simulink model "KeplerianPropagator_Basic"  (R2017b)
settings: Solver=ode3  StartTime=0.0  StopTime=stopTime  FixedStep=stepSize  MaxStep=100  RelTol=1e-3  EnableMultiTasking=on
values from neighbouring files (symbols this model uses):
  a = a_d    (= 6782.423)    [AA279D_hw4.m]    (also in AA279D_hw4_v2.m = 7500; SCHAUBprop.m = oe(1); TLE_Reader.m = (mu/n^2)^(1/3); keplerUniversal.m = 1./alpha(idx))
  e = 0    [AA279D_PSET3.m]    (also in AA279D_PSET4.m = 0.1; AA279D_hw4.m = 0.7; AA279D_hw4_v2.m = 0.1; SCHAUBprop.m = oe(2))
  i = i_d    [AA279D_hw4.m]    (also in SCHAUBprop.m = oe(3); dv_hardcod.m = cin+1; dv_timer.m = cin+1; oe2roe.m = oe_c(3))
  M0 = M    [AA279D_FINAL.m]    (also in AA279D_PSET1.m; AA279D_PSET2.m; AA279D_PSET2_a_change.m; AA279D_PSET3.m)
  n = n_D    [AA279D_hw4.m]    (also in AA279D_hw4_v2.m = sqrt(mu/a^3); AA279D_hw5_dv.m = sqrt(mu/at^3); OE2ECI.m = sqrt(mu/a^3); TLE_Reader.m = revs_per_day*2*pi/(24*3600))
  RAAN = 0    [AA279D_FINAL.m]    (also in AA279D_hw4_v2.m = deg2rad(358.1559); TLE_Reader.m = L3(1,4); test_space.mat = 331.1221)
  tol = 10^-5    (= 1e-05)    [AA279D_FINAL.m]    (also in AA279D_PSET1.m; AA279D_PSET2.m; AA279D_PSET2_a_change.m; AA279D_PSET3.m)
  w = 0    [AA279D_FINAL.m]    (also in AA279D_hw4.m = w_d; AA279D_hw4_v2.m = deg2rad(358.729); SCHAUBprop.m = oe(5); TLE_Reader.m = L3(1,6))
libraries: simulink_extras x4
settings Model: Creator=Lloyd  LastModifiedBy=cwcovert
settings DataIOCC: LimitDataPoints=on  SaveFormat=Array
settings OptimizationCC: LifeSpan=inf
settings DebuggingCC: SolverPrmCheckMsg=warning  SFUnexpectedBacktrackingDiag=warning  SFNoUnconditionalDefaultTransitionDiag=warning  SFExecutionAtInitializationDiag=none
settings HardwareCC: ProdBitPerPointer=32  ProdBitPerSizeT=32  ProdBitPerPtrDiffT=32  ProdLargestAtomicFloat=None  ProdIntDivRoundTo=Undefined  ProdEndianess=Unspecified  ProdWordSize=32  ProdHWDeviceType=32-bit Generic
settings ModelReferenceCC: PropagateSignalLabelsOutOfModel=off
settings CodeAppCC: StateflowObjectComments=on
settings GRTTargetCC: TargetLangStandard=C89/C90 (ANSI)  GeneratePreprocessorConditionals=Disable all
settings ConfigComp: CovMetricSettings=dw  CovHtmlReporting=on  CovSaveCumulativeToWorkspaceVar=on  CovSaveSingleToWorkspaceVar=on  CovExternalEMLEnable=off  CovSFcnEnable=off

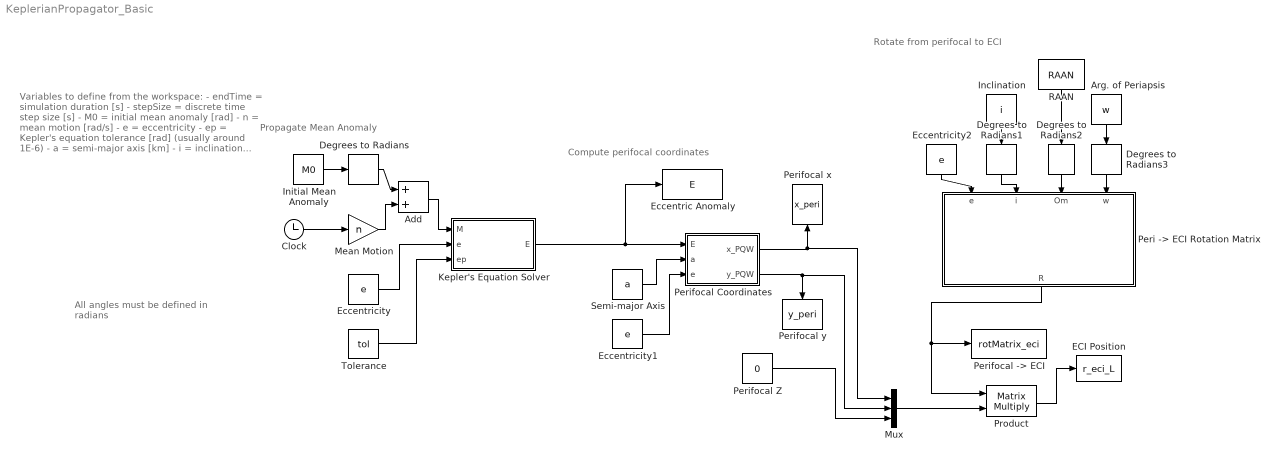
== system KeplerianPropagator_Basic ==
  note: Rotate from perifocal to ECI
  note: Compute perifocal coordinates
  note: Propagate Mean Anomaly
  note: All angles must be defined in radians
  note: Variables to define from the workspace:
      |
      | - endTime = simulation duration [s]
      | - stepSize = discrete time step size [s]
      |
      | - M0 = initial mean anomaly [rad]
      | - n = mean motion [rad/s]
      | - e = eccentricity
      | - ep = Kepler's equation tolerance [rad] (usually around 1E-6)
      |
      | - a = semi-major axis [km]
      | - i = inclination [rad]
      | - Om = RAAN [rad]
      | - w = arg. of peri. [rad]
  Add : Sum
  Arg. of Periapsis : Constant  Value=w
  Clock : Clock
  Degrees to Radians{,1..3} (4 alike) : simulink_extras/Transformations/Degrees to Radians
  ECI Position : ToWorkspace  VariableName=r_eci_L  SampleTime=-1
  Eccentric Anomaly : ToWorkspace  VariableName=E  SampleTime=-1
  Eccentricity : Constant  Value=e
  Eccentricity1 : Constant  Value=e
  Eccentricity2 : Constant  Value=e
  Inclination : Constant  Value=i
  Initial Mean Anomaly : Constant  Value=M0
  Kepler's Equation Solver : MATLAB Function  TreatAsAtomicUnit=on
  Mean Motion : Gain  Gain=n
  Mux : Mux  Inputs=3
  "Peri -> ECI Rotation Matrix" : MATLAB Function  TreatAsAtomicUnit=on
  "Perifocal -> ECI" : ToWorkspace  VariableName=rotMatrix_eci  SaveFormat=Structure  SampleTime=-1
  Perifocal Coordinates : MATLAB Function  TreatAsAtomicUnit=on
  Perifocal Z : Constant  Value=0
  Perifocal x : ToWorkspace  VariableName=x_peri  SampleTime=-1
  Perifocal y : ToWorkspace  VariableName=y_peri  SampleTime=-1
  Product : Product  Multiplication=Matrix(*)
  RAAN : Constant  Value=RAAN
  Semi-major Axis : Constant  Value=a
  Tolerance : Constant  Value=tol
  wires:
  Clock/1 -> Mean Motion/1
  Mean Motion/1 -> Add/2
  Eccentricity/1 -> Kepler's Equation Solver/2(e)
  Tolerance/1 -> Kepler's Equation Solver/3(ep)
  Add/1 -> Kepler's Equation Solver/1(M)
  Mux/1 -> Product/2
  Perifocal Z/1 -> Mux/3
  "Peri -> ECI Rotation Matrix"/1(R) -> "Perifocal -> ECI"/1, Product/1
  Product/1 -> ECI Position/1
  Perifocal Coordinates/2(y_PQW) -> Mux/2, Perifocal y/1
  Perifocal Coordinates/1(x_PQW) -> Mux/1, Perifocal x/1
  Kepler's Equation Solver/1(E) -> Perifocal Coordinates/1(E), Eccentric Anomaly/1
  Eccentricity1/1 -> Perifocal Coordinates/3(e)
  Semi-major Axis/1 -> Perifocal Coordinates/2(a)
  RAAN/1 -> Degrees to Radians2/1
  Arg. of Periapsis/1 -> Degrees to Radians3/1
  Inclination/1 -> Degrees to Radians1/1
  Eccentricity2/1 -> "Peri -> ECI Rotation Matrix"/1(e)
  Initial Mean Anomaly/1 -> Degrees to Radians/1
  Degrees to Radians/1 -> Add/1
  Degrees to Radians1/1 -> "Peri -> ECI Rotation Matrix"/2(i)
  Degrees to Radians2/1 -> "Peri -> ECI Rotation Matrix"/3(Om)
  Degrees to Radians3/1 -> "Peri -> ECI Rotation Matrix"/4(w)

== matlab function KeplerianPropagator_Basic/Kepler's Equation Solver ==
  data: M input; E output; e input; ep input
function E = keplerEq(M, e, ep)
% keplersEquationSolver solves Kepler's equation for an eccentric anomaly
% given a mean anomaly value, orbit eccentricity, and a tolerance.

% Check for valid inputs
if (e < 0) || (e >= 1)
    error('Please provide an eccentricity corresponding to a closed orbit (0 < e < 1)');
end

if M == 0 || M == pi
    % Return the known solutions (trivial)
    E = M;
else
    % Set up the problem based on an initial guess
    E0 = M;
    d = -(E0 - e*sin(E0) - M)/(1 - e*cos(E0));
    
    % Loop until the solution converges
    while abs(d) > ep
        E1 = E0 + d;
        
        d = -(E1 - e*sin(E1) - M)/(1 - e*cos(E1));
        
        E0 = E1;
    end
    
    E = E0;
end

% if M == 0
%     E_i1 = pi;
% else
%     E_i1 = M;
% end
% 
% fE_i1 = E_i1 - e*sin(E_i1) - M;
% fE_i1_p = 1 - e*cos(E_i1);
% 
% di = -fE_i1/fE_i1_p;
% 
% while abs(di) > ep
%     E_i2 = E_i1 + di;
%     
%     fE_i = E_i2 - e*sin(E_i2) - M;
%     fE_i_p = 1 - e*cos(E_i2);
%     
%     di = -fE_i/fE_i_p;
%     E_i1 = E_i2;
% end
% 
% E = E_i1;

end

== matlab function KeplerianPropagator_Basic/Perifocal Coordinates ==
  data: E input; a input; x_PQW output; e input; y_PQW output
function [x_PQW, y_PQW] = E2Pos(E, a, e)

% Compute position in perifocal coordinates
%
% Inputs
% ------
% E         Eccentric anomaly
% a         semi-major axis
%
% Outputs
% -------
% x         x position on orbital plane
% y         y position on orbital plane

% semi-latus rectum
p = a*(1 - e^2);

% Compute true anomaly from eccentric anomaly
cos_nu = (cos(E) - e) / (1 - e*cos(E));
sin_nu = (sin(E)*sqrt(1 - e^2)) / (1 - e*cos(E));
nu = atan2(sin_nu, cos_nu);

% Compute radial position
r = p / (1 + e*cos(nu));

% convert to cartesian
x_PQW = r*cos(nu);
y_PQW = r*sin(nu);

== matlab function KeplerianPropagator_Basic/Peri -> ECI Rotation Matrix ==
  data: e input; R output; i input; Om input; w input
function R = rotPeri2ECI(e, i, Om, w)

RzOm = [ cos(-Om), sin(-Om), 0;
        -sin(-Om), cos(-Om), 0;
                0,        0, 1];
            
Rxi = [1,        0,       0;
       0,  cos(-i), sin(-i);
       0, -sin(-i), cos(-i)];
   
Rzw= [ cos(-w), sin(-w), 0;
        -sin(-w), cos(-w), 0;
               0,       0, 1];

R = RzOm*Rxi*Rzw;

if i == 0 && e ~= 0         % Equatorial + elliptical
    R = Rzw;
elseif e == 0 && i ~= 0     % Circular + inclined
    R = RzOm*Rxi;
elseif i == 0 && e == 0     % Equatorial + circular
    R = eye(3);    
end
